simulink library "relay_bkrCtrl_lib"  (Simulink 8.1)
settings: Solver=ode45  StartTime=0.0  StopTime=10.0  RelTol=1e-3
undefined symbols (not defined in the file): bkrCtrl_enable, bkrCtrl_status, Ts
settings Model: Creator=RE25624  LastModifiedBy=RE25624

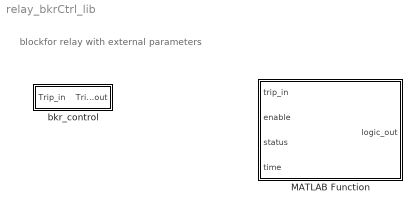
== system relay_bkrCtrl_lib ==
  note: blockfor relay with external parameters
  MATLAB Function : MATLAB Function  TreatAsAtomicUnit=on
  bkr_control : Subsystem  mask(Breaker control){enable=bkrCtrl_enable, status=bkrCtrl_status}
      mask prompts: status "Breaker status: [1-closed, 0-open]"
      mask help: Allows the user to select which trip signal will be received at the breaker.

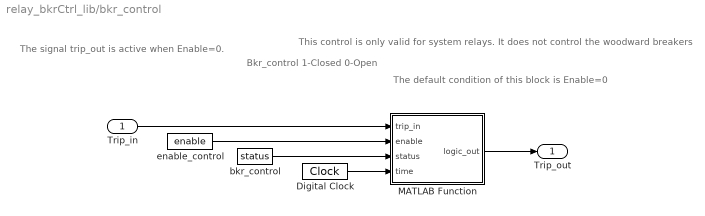
== system relay_bkrCtrl_lib/bkr_control ==
  note: The signal trip_out is active when Enable=0.
  note: Bkr_control
      | 1-Closed
      | 0-Open
  note: This control is only valid for system relays.
      | It does not control the woodward breakers
  note: The default condition of this block is Enable=0
  Trip_in : Inport
  Digital Clock : DigitalClock  SampleTime=Ts
  MATLAB Function : MATLAB Function  TreatAsAtomicUnit=on
  bkr_control : Constant  Value=status
  enable_control : Constant  Value=enable
  Trip_out : Outport
  wires:
  Digital Clock/1 -> MATLAB Function/4(time)
  bkr_control/1 -> MATLAB Function/3(status)
  enable_control/1 -> MATLAB Function/2(enable)
  Trip_in/1 -> MATLAB Function/1(trip_in)
  MATLAB Function/1(logic_out) -> Trip_out/1

== matlab function bkr_control/MATLAB Function ==
  data: trip_in input double; logic_out output double; enable input double; status input double; time input double
% CREATED BY: REYNALDO SALCEDO
% LAST CHANGE BY : REYNALDO SALCEDO
% GROUP: 73
% DATE MODIFIED  : 04/13/2016
%

function logic_out = fcn(trip_in, enable, status, time)
%#codegen

t_logic = 0.3; % time [sec] to activate logic
if enable == 1
    logic_out = status;
else
    if time > t_logic
        logic_out = trip_in;
    else
        logic_out = 1;
    end
end

== matlab function MATLAB Function ==
  data: trip_in input double; logic_out output double; enable input double; status input double; time input double
% CREATED BY: REYNALDO SALCEDO
% LAST CHANGE BY : REYNALDO SALCEDO
% GROUP: 73
% DATE MODIFIED  : 04/13/2016
%

function logic_out = fcn(trip_in, enable, status, time)
%#codegen

t_logic = 0.3; % time [sec] to activate logic
if enable == 1
    logic_out = status;
else
    if time > t_logic
        logic_out = trip_in;
    else
        logic_out = 1;
    end
end
